simulink model "L11Model"  (R2020b)
settings: Solver=VariableStepAuto  StartTime=0.0  StopTime=10000.0  RelTol=1e-3
values from neighbouring files (symbols this model uses):
  a = 0.99    [L11.m]
settings Model: Creator=Nic  LastModifiedBy=Nic

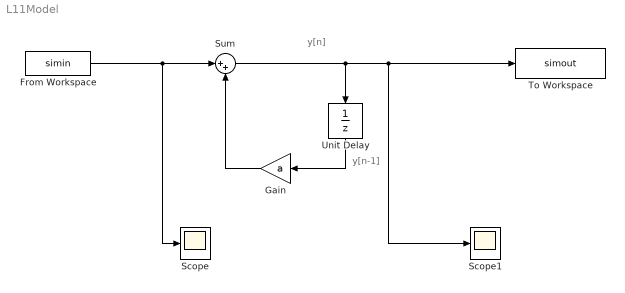
== system L11Model ==
  note: y[n-1]
  note: y[n]
  From Workspace : FromWorkspace  VariableName=simin  SampleTime=1
  Gain : Gain  Gain=a
  Scope : Scope
  Scope1 : Scope
  Sum : Sum  Inputs=|++
  To Workspace : ToWorkspace  VariableName=simout  SampleTime=-1
  Unit Delay : UnitDelay  SampleTime=-1  HasFrameUpgradeWarning=on
  wires:
  Sum/1 -> Scope1/1, To Workspace/1, Unit Delay/1
  Unit Delay/1 -> Gain/1
  Gain/1 -> Sum/2
  From Workspace/1 -> Scope/1, Sum/1
